simulink model "Electric"  (R2022b)
settings: Solver=VariableStepAuto  StartTime=0.0  StopTime=2  RelTol=1e-3
settings Model: Creator=Stefano  LastModifiedBy=stefanopanzieri
settings SolverCC: AlgebraicLoopSolver=TrustRegion
settings DebuggingCC: UnconnectedInputMsg=warning  UnconnectedOutputMsg=warning  UnconnectedLineMsg=warning  SFMachineParentedDataDiag=warning
settings ModelReferenceCC: EnableRefExpFcnMdlSchedulingChecks=on
settings SFSimCC: CustomCodeUndefinedFunction=UseInterfaceOnly
settings RTWCC: DLArmComputeVersion=19.05

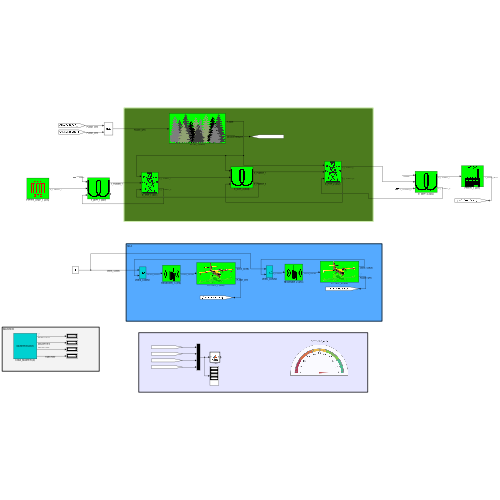
[thumbnail: Simulink's stored preview of the top-level diagram]
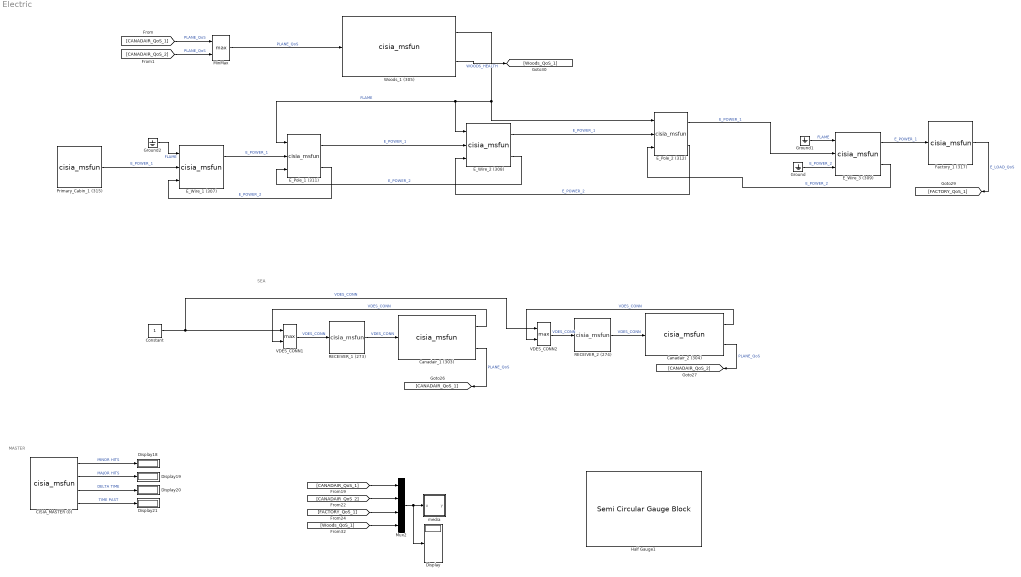
== system Electric ==
  note: SEA
  note: MASTER
  CISIA_MASTER (0) : M-S-Function  FunctionName=cisia_msfun  Parameters=Parameter1, Parameter2, Parameter3, resources, Parameter4, Parameter5, Parameter6, Parameter7, Parameter8, Parameter9,Parameter11  mask(S-function:msfcn_unit_delay){Parameter1='CISIA_MASTER', Parameter2=1, Parameter3='SistemiIoT', resources=off, Parameter4=on, Parameter5=off, Parameter6=off, Parameter7=off, Parameter8=0.001, Parameter9=off, Parameter11=on}
      mask prompts: Parameter1 "entity name"; Parameter2 "sampling time"; Parameter3 "project"; resources "Save status at each major hit"; Parameter4 "Show Operative Levels with colors"; Parameter5 "Load Entities from file"; Parameter6 "Load Start from Mask"; Parameter7 "Real Time"; Parameter8 "Real Time Hit (sec)"; Parameter9 "Skip saving"; Parameter11 "Show unconnected"
      mask help: This is a level-2 MATLAB file S-function which demonstrates CISIA entity
      mask Display: disp('MASTER BLOCK')
  Canadair_1 (303) : M-S-Function  FunctionName=cisia_msfun  Parameters=Parameter1, Parameter2, Parameter3, resources, Parameter10, codeupdate, step_received, step_computed, dynamic_computed, step_sended, id_entity, id_project, id_type, name_type, color  mask(S-function:msfcn_unit_delay){Parameter1='Canadair_1', Parameter2=1, Parameter3='', resources=|, Parameter10=off, codeupdate=off, step_received=|, step_computed=, dynamic_computed=, step_sended=|, id_entity=303, id_project=6, id_type=64, name_type=Plane, color=#FFFFFF}
      mask resources=|
      | *** INPUT RESOURCES ***
      | NUM_INPUTS 1
      | VDES_CONN (1)
      |
      | *** STATE VARIABLES ***
      | NUM_VARIABLES 3
      | Operative_Level(NUMERIC)(1)(1)
      | Mechanical_Fault(NUMERIC)(1)(0)
      | Conn_Fault(NUMERIC)(1)(0)
      |
      | *** OUTPUT RESOURCES ***
      | NUM_OUTPUTS 2
      | VDES_CONN (1)
      | PLANE_QoS (1)
      mask step_received=|
      | Conn_Fault=1-max(VDES_CONN);
      |
      |
      | Operative_Level=(1-Mechanical_Fault)*(1-Conn_Fault);
      mask step_sended=|
      | PLANE_QoS=Operative_Level;
      | VDES_CONN=1-Conn_Fault;
      mask prompts: Parameter1 "entity name"; Parameter2 "sampling time"; Parameter3 "project"; resources "input resources and state variables"; Parameter10 "Bring state variables to output"; codeupdate "update code from mask"
      mask help: This is a level-2 MATLAB file S-function which demonstrates CISIA entity
      mask DialogControl Container1 Prompt: All parameters
      mask Display: image('Icons/Canadair_1.png')
  Canadair_2 (304) : M-S-Function  FunctionName=cisia_msfun  Parameters=Parameter1, Parameter2, Parameter3, resources, Parameter10, codeupdate, step_received, step_computed, dynamic_computed, step_sended, id_entity, id_project, id_type, name_type, color  mask(S-function:msfcn_unit_delay){Parameter1='Canadair_2', Parameter2=1, Parameter3='', resources=|, Parameter10=off, codeupdate=off, step_received=|, step_computed=, dynamic_computed=, step_sended=|, id_entity=304, id_project=6, id_type=64, name_type=Plane, color=#FFFFFF}
      mask resources=|
      | *** INPUT RESOURCES ***
      | NUM_INPUTS 1
      | VDES_CONN (1)
      |
      | *** STATE VARIABLES ***
      | NUM_VARIABLES 3
      | Operative_Level(NUMERIC)(1)(1)
      | Mechanical_Fault(NUMERIC)(1)(0)
      | Conn_Fault(NUMERIC)(1)(0)
      |
      | *** OUTPUT RESOURCES ***
      | NUM_OUTPUTS 2
      | VDES_CONN (1)
      | PLANE_QoS (1)
      mask step_received=|
      | Conn_Fault=1-max(VDES_CONN);
      |
      |
      | Operative_Level=(1-Mechanical_Fault)*(1-Conn_Fault);
      mask step_sended=|
      | PLANE_QoS=Operative_Level;
      | VDES_CONN=1-Conn_Fault;
      mask prompts: Parameter1 "entity name"; Parameter2 "sampling time"; Parameter3 "project"; resources "input resources and state variables"; Parameter10 "Bring state variables to output"; codeupdate "update code from mask"
      mask help: This is a level-2 MATLAB file S-function which demonstrates CISIA entity
      mask DialogControl Container1 Prompt: All parameters
      mask Display: image('Icons/Canadair_2.png')
  Constant : Constant
  Display{,18..21} (5 alike) : Display
  E_Pole_1 (311) : M-S-Function  FunctionName=cisia_msfun  Parameters=Parameter1, Parameter2, Parameter3, resources, Parameter10, codeupdate, step_received, step_computed, dynamic_computed, step_sended, id_entity, id_project, id_type, name_type, color  mask(S-function:msfcn_unit_delay){Parameter1='E_Pole_1', Parameter2=1, Parameter3='', resources=|, Parameter10=off, codeupdate=off, step_received=|, step_computed=, dynamic_computed=, step_sended=|, id_entity=311, id_project=6, id_type=68, name_type=Electric_Pole, color=#FFFFFF}
      mask resources=|
      | *** INPUT RESOURCES ***
      | NUM_INPUTS 3
      | FLAME (1)
      | E_POWER_1 (10)
      | E_POWER_2 (10)
      |
      | *** STATE VARIABLES ***
      | NUM_VARIABLES 5
      | Operative_Level(NUMERIC)(1)(1)
      | Mechanical_Fault(NUMERIC)(1)(0)
      | Fire_Fault(NUMERIC)(1)(0)
      | Physical_Fault(NUMERIC)(1)(0)
      | Power_Gen(NUMERIC_ARRAY)(10)(0  0  0  0  0  0  0  0  0  0)
      |
      | *** OUTPUT RESOURCES ***
      | NUM_OUTPUTS 2
      | E_POWER_1 (10)
      | E_POWER_2 (10)
      mask step_received=|
      | Power_Gen=max(E_POWER_1,E_POWER_2);
      |
      | Fire_Fault=FLAME;
      |
      | Physical_Fault=max(Fire_Fault,Mechanical_Fault);
      |
      | Operative_Level=1-Physical_Fault;
      mask step_sended=|
      | E_POWER_1=Power_Gen*(1-Physical_Fault);
      | E_POWER_2=Power_Gen*(1-Physical_Fault);
      mask prompts: Parameter1 "entity name"; Parameter2 "sampling time"; Parameter3 "project"; resources "input resources and state variables"; Parameter10 "Bring state variables to output"; codeupdate "update code from mask"
      mask help: This is a level-2 MATLAB file S-function which demonstrates CISIA entity
      mask DialogControl Container1 Prompt: All parameters
      mask Display: image('Icons/Electric_Pole.png')
  E_Pole_2 (312) : M-S-Function  FunctionName=cisia_msfun  Parameters=Parameter1, Parameter2, Parameter3, resources, Parameter10, codeupdate, step_received, step_computed, dynamic_computed, step_sended, id_entity, id_project, id_type, name_type, color  mask(S-function:msfcn_unit_delay){Parameter1='E_Pole_2', Parameter2=1, Parameter3='', resources=|, Parameter10=off, codeupdate=off, step_received=|, step_computed=, dynamic_computed=, step_sended=|, id_entity=312, id_project=6, id_type=68, name_type=Electric_Pole, color=#FFFFFF}
      mask resources=|
      | *** INPUT RESOURCES ***
      | NUM_INPUTS 3
      | FLAME (1)
      | E_POWER_1 (10)
      | E_POWER_2 (10)
      |
      | *** STATE VARIABLES ***
      | NUM_VARIABLES 5
      | Operative_Level(NUMERIC)(1)(1)
      | Mechanical_Fault(NUMERIC)(1)(0)
      | Fire_Fault(NUMERIC)(1)(0)
      | Physical_Fault(NUMERIC)(1)(0)
      | Power_Gen(NUMERIC_ARRAY)(10)(0  0  0  0  0  0  0  0  0  0)
      |
      | *** OUTPUT RESOURCES ***
      | NUM_OUTPUTS 2
      | E_POWER_1 (10)
      | E_POWER_2 (10)
      mask step_received=|
      | Power_Gen=max(E_POWER_1,E_POWER_2);
      |
      | Fire_Fault=FLAME;
      |
      | Physical_Fault=max(Fire_Fault,Mechanical_Fault);
      |
      | Operative_Level=1-Physical_Fault;
      mask step_sended=|
      | E_POWER_1=Power_Gen*(1-Physical_Fault);
      | E_POWER_2=Power_Gen*(1-Physical_Fault);
      mask prompts: Parameter1 "entity name"; Parameter2 "sampling time"; Parameter3 "project"; resources "input resources and state variables"; Parameter10 "Bring state variables to output"; codeupdate "update code from mask"
      mask help: This is a level-2 MATLAB file S-function which demonstrates CISIA entity
      mask DialogControl Container1 Prompt: All parameters
      mask Display: image('Icons/Electric_Pole.png')
  E_Wire_1 (307) : M-S-Function  FunctionName=cisia_msfun  Parameters=Parameter1, Parameter2, Parameter3, resources, Parameter10, codeupdate, step_received, step_computed, dynamic_computed, step_sended, id_entity, id_project, id_type, name_type, color  mask(S-function:msfcn_unit_delay){Parameter1='E_Wire_1', Parameter2=1, Parameter3='', resources=|, Parameter10=off, codeupdate=off, step_received=|, step_computed=, dynamic_computed=, step_sended=|, id_entity=307, id_project=6, id_type=67, name_type=Electric_Wire, color=#FFFFFF}
      mask resources=|
      | *** INPUT RESOURCES ***
      | NUM_INPUTS 3
      | FLAME (1)
      | E_POWER_1 (10)
      | E_POWER_2 (10)
      |
      | *** STATE VARIABLES ***
      | NUM_VARIABLES 5
      | Operative_Level(NUMERIC)(1)(1)
      | Mechanical_Fault(NUMERIC)(1)(0)
      | Fire_Fault(NUMERIC)(1)(0)
      | Physical_Fault(NUMERIC)(1)(0)
      | Power_Gen(NUMERIC_ARRAY)(10)(0  0  0  0  0  0  0  0  0  0)
      |
      | *** OUTPUT RESOURCES ***
      | NUM_OUTPUTS 2
      | E_POWER_1 (10)
      | E_POWER_2 (10)
      mask step_received=|
      | Power_Gen=max(E_POWER_1,E_POWER_2);
      |
      | Fire_Fault=FLAME;
      |
      | Physical_Fault=max(Fire_Fault,Mechanical_Fault);
      |
      | Operative_Level=1-Physical_Fault;
      mask step_sended=|
      | E_POWER_1=Power_Gen*(1-Physical_Fault);
      | E_POWER_2=Power_Gen*(1-Physical_Fault);
      mask prompts: Parameter1 "entity name"; Parameter2 "sampling time"; Parameter3 "project"; resources "input resources and state variables"; Parameter10 "Bring state variables to output"; codeupdate "update code from mask"
      mask help: This is a level-2 MATLAB file S-function which demonstrates CISIA entity
      mask DialogControl Container1 Prompt: All parameters
      mask Display: image('Icons/Electric_Wire.png')
  E_Wire_2 (308) : M-S-Function  FunctionName=cisia_msfun  Parameters=Parameter1, Parameter2, Parameter3, resources, Parameter10, codeupdate, step_received, step_computed, dynamic_computed, step_sended, id_entity, id_project, id_type, name_type, color  mask(S-function:msfcn_unit_delay){Parameter1='E_Wire_2', Parameter2=1, Parameter3='', resources=|, Parameter10=off, codeupdate=off, step_received=|, step_computed=, dynamic_computed=, step_sended=|, id_entity=308, id_project=6, id_type=67, name_type=Electric_Wire, color=#FFFFFF}
      mask resources=|
      | *** INPUT RESOURCES ***
      | NUM_INPUTS 3
      | FLAME (1)
      | E_POWER_1 (10)
      | E_POWER_2 (10)
      |
      | *** STATE VARIABLES ***
      | NUM_VARIABLES 5
      | Operative_Level(NUMERIC)(1)(1)
      | Mechanical_Fault(NUMERIC)(1)(0)
      | Fire_Fault(NUMERIC)(1)(0)
      | Physical_Fault(NUMERIC)(1)(0)
      | Power_Gen(NUMERIC_ARRAY)(10)(0  0  0  0  0  0  0  0  0  0)
      |
      | *** OUTPUT RESOURCES ***
      | NUM_OUTPUTS 2
      | E_POWER_1 (10)
      | E_POWER_2 (10)
      mask step_received=|
      | Power_Gen=max(E_POWER_1,E_POWER_2);
      |
      | Fire_Fault=FLAME;
      |
      | Physical_Fault=max(Fire_Fault,Mechanical_Fault);
      |
      | Operative_Level=1-Physical_Fault;
      mask step_sended=|
      | E_POWER_1=Power_Gen*(1-Physical_Fault);
      | E_POWER_2=Power_Gen*(1-Physical_Fault);
      mask prompts: Parameter1 "entity name"; Parameter2 "sampling time"; Parameter3 "project"; resources "input resources and state variables"; Parameter10 "Bring state variables to output"; codeupdate "update code from mask"
      mask help: This is a level-2 MATLAB file S-function which demonstrates CISIA entity
      mask DialogControl Container1 Prompt: All parameters
      mask Display: image('Icons/Electric_Wire.png')
  E_Wire_3 (309) : M-S-Function  FunctionName=cisia_msfun  Parameters=Parameter1, Parameter2, Parameter3, resources, Parameter10, codeupdate, step_received, step_computed, dynamic_computed, step_sended, id_entity, id_project, id_type, name_type, color  mask(S-function:msfcn_unit_delay){Parameter1='E_Wire_3', Parameter2=1, Parameter3='', resources=|, Parameter10=off, codeupdate=off, step_received=|, step_computed=, dynamic_computed=, step_sended=|, id_entity=309, id_project=6, id_type=67, name_type=Electric_Wire, color=#FFFFFF}
      mask resources=|
      | *** INPUT RESOURCES ***
      | NUM_INPUTS 3
      | FLAME (1)
      | E_POWER_1 (10)
      | E_POWER_2 (10)
      |
      | *** STATE VARIABLES ***
      | NUM_VARIABLES 5
      | Operative_Level(NUMERIC)(1)(1)
      | Mechanical_Fault(NUMERIC)(1)(0)
      | Fire_Fault(NUMERIC)(1)(0)
      | Physical_Fault(NUMERIC)(1)(0)
      | Power_Gen(NUMERIC_ARRAY)(10)(0  0  0  0  0  0  0  0  0  0)
      |
      | *** OUTPUT RESOURCES ***
      | NUM_OUTPUTS 2
      | E_POWER_1 (10)
      | E_POWER_2 (10)
      mask step_received=|
      | Power_Gen=max(E_POWER_1,E_POWER_2);
      |
      | Fire_Fault=FLAME;
      |
      | Physical_Fault=max(Fire_Fault,Mechanical_Fault);
      |
      | Operative_Level=1-Physical_Fault;
      mask step_sended=|
      | E_POWER_1=Power_Gen*(1-Physical_Fault);
      | E_POWER_2=Power_Gen*(1-Physical_Fault);
      mask prompts: Parameter1 "entity name"; Parameter2 "sampling time"; Parameter3 "project"; resources "input resources and state variables"; Parameter10 "Bring state variables to output"; codeupdate "update code from mask"
      mask help: This is a level-2 MATLAB file S-function which demonstrates CISIA entity
      mask DialogControl Container1 Prompt: All parameters
      mask Display: image('Icons/Electric_Wire.png')
  Factory_1 (317) : M-S-Function  FunctionName=cisia_msfun  Parameters=Parameter1, Parameter2, Parameter3, resources, Parameter10, codeupdate, step_received, step_computed, dynamic_computed, step_sended, id_entity, id_project, id_type, name_type, color  mask(S-function:msfcn_unit_delay){Parameter1='Factory_1', Parameter2=1, Parameter3='', resources=|, Parameter10=off, codeupdate=off, step_received=|, step_computed=, dynamic_computed=, step_sended=E_LOAD_QoS=Operative_Level;, id_entity=317, id_project=6, id_type=69, name_type=Electric_Load, color=#FFFFFF}
      mask resources=|
      | *** INPUT RESOURCES ***
      | NUM_INPUTS 1
      | E_POWER_1 (10)
      |
      | *** STATE VARIABLES ***
      | NUM_VARIABLES 7
      | Operative_Level(NUMERIC)(1)(1)
      | Mechanical_Fault(NUMERIC)(1)(0)
      | Power_Fault(NUMERIC)(1)(0)
      | Fire_Fault(NUMERIC)(1)(0)
      | Physical_Fault(NUMERIC)(1)(0)
      | Power_Gen(NUMERIC_ARRAY)(10)(0  0  0  0  0  0  0  0  0  0)
      | Consumed_Power(NUMERIC_ARRAY)(10)(0  0  0  0  0  0  0  0  0  0)
      |
      | *** OUTPUT RESOURCES ***
      | NUM_OUTPUTS 1
      | E_LOAD_QoS (1)
      mask step_received=|
      | Power_Gen=max(Power_Gen_init,E_POWER_1);
      |
      | Physical_Fault=max([Fire_Fault  Mechanical_Fault] );
      |
      | Power_Fault=max(abs(Consumed_Power.*E_POWER_1-Consumed_Power));
      |
      |
      | Operative_Level=max([1-Power_Fault 0.5])*(1-Physical_Fault);
      mask prompts: Parameter1 "entity name"; Parameter2 "sampling time"; Parameter3 "project"; resources "input resources and state variables"; Parameter10 "Bring state variables to output"; codeupdate "update code from mask"
      mask help: This is a level-2 MATLAB file S-function which demonstrates CISIA entity
      mask DialogControl Container1 Prompt: All parameters
      mask Display: image('Icons/Factory_1.png')
  Ground : Ground
  Ground1 : Ground
  Ground2 : Ground
  Half Gauge1 : SemiCircularGaugeBlock  ScaleMax=1
  MinMax : MinMax  Function=max  Inputs=2
  Mux2 : Mux
  Primary_Cabin_1 (315) : M-S-Function  FunctionName=cisia_msfun  Parameters=Parameter1, Parameter2, Parameter3, resources, Parameter10, codeupdate, step_received, step_computed, dynamic_computed, step_sended, id_entity, id_project, id_type, name_type, color  mask(S-function:msfcn_unit_delay){Parameter1='Primary_Cabin_1', Parameter2=1, Parameter3='', resources=|, Parameter10=off, codeupdate=off, step_received=|, step_computed=, dynamic_computed=, step_sended=E_POWER_1=Power_Gen*(1-Physical_Fault);, id_entity=315, id_project=6, id_type=66, name_type=Electric_Plant, color=#FFFFFF}
      mask resources=|
      | *** INPUT RESOURCES ***
      | NUM_INPUTS 0
      |
      | *** STATE VARIABLES ***
      | NUM_VARIABLES 5
      | Operative_Level(NUMERIC)(1)(1)
      | Mechanical_Fault(NUMERIC)(1)(0)
      | Fire_Fault(NUMERIC)(1)(0)
      | Physical_Fault(NUMERIC)(1)(0)
      | Power_Gen(NUMERIC_ARRAY)(10)(0  0  0  0  0  0  0  0  0  0)
      |
      | *** OUTPUT RESOURCES ***
      | NUM_OUTPUTS 1
      | E_POWER_1 (10)
      mask step_received=|
      | Physical_Fault=max(Fire_Fault,Mechanical_Fault);
      |
      | Operative_Level=1-Physical_Fault;
      mask prompts: Parameter1 "entity name"; Parameter2 "sampling time"; Parameter3 "project"; resources "input resources and state variables"; Parameter10 "Bring state variables to output"; codeupdate "update code from mask"
      mask help: This is a level-2 MATLAB file S-function which demonstrates CISIA entity
      mask DialogControl Container1 Prompt: All parameters
      mask Display: image('Icons/Primary_Cabin_1.png')
  RECEIVER_1 (273) : M-S-Function  FunctionName=cisia_msfun  Parameters=Parameter1, Parameter2, Parameter3, resources, Parameter10, codeupdate, step_received, step_computed, dynamic_computed, step_sended, id_entity, id_project, id_type, name_type, color  mask(S-function:msfcn_unit_delay){Parameter1='RECEIVER_1', Parameter2=1, Parameter3='', resources=|, Parameter10=off, codeupdate=off, step_received=Conn_Fault=1-VDES_CONN;, step_computed=, dynamic_computed=, step_sended=VDES_CONN=1-Conn_Fault;, id_entity=273, id_project=6, id_type=59, name_type=VDES_RECEIVER, color=#FFFFFF}
      mask resources=|
      | *** INPUT RESOURCES ***
      | NUM_INPUTS 1
      | VDES_CONN (1)
      |
      | *** STATE VARIABLES ***
      | NUM_VARIABLES 3
      | Operative_Level(NUMERIC)(1)(1)
      | Connection(NUMERIC_ARRAY)(20)(0  0  0  0  0  0  0  0  0  0  0  0  0  0  0  0  0  0  0  0)
      | Conn_Fault(NUMERIC)(1)(0)
      |
      | *** OUTPUT RESOURCES ***
      | NUM_OUTPUTS 1
      | VDES_CONN (1)
      mask prompts: Parameter1 "entity name"; Parameter2 "sampling time"; Parameter3 "project"; resources "input resources and state variables"; Parameter10 "Bring state variables to output"; codeupdate "update code from mask"
      mask help: This is a level-2 MATLAB file S-function which demonstrates CISIA entity
      mask DialogControl Container1 Prompt: All parameters
      mask Display: image('Icons/VDES_RECEIVER.png')
  RECEIVER_2 (274) : M-S-Function  FunctionName=cisia_msfun  Parameters=Parameter1, Parameter2, Parameter3, resources, Parameter10, codeupdate, step_received, step_computed, dynamic_computed, step_sended, id_entity, id_project, id_type, name_type, color  mask(S-function:msfcn_unit_delay){Parameter1='RECEIVER_2', Parameter2=1, Parameter3='', resources=|, Parameter10=off, codeupdate=off, step_received=Conn_Fault=1-VDES_CONN;, step_computed=, dynamic_computed=, step_sended=VDES_CONN=1-Conn_Fault;, id_entity=274, id_project=6, id_type=59, name_type=VDES_RECEIVER, color=#FFFFFF}
      mask resources=|
      | *** INPUT RESOURCES ***
      | NUM_INPUTS 1
      | VDES_CONN (1)
      |
      | *** STATE VARIABLES ***
      | NUM_VARIABLES 3
      | Operative_Level(NUMERIC)(1)(1)
      | Connection(NUMERIC_ARRAY)(20)(0  0  0  0  0  0  0  0  0  0  0  0  0  0  0  0  0  0  0  0)
      | Conn_Fault(NUMERIC)(1)(0)
      |
      | *** OUTPUT RESOURCES ***
      | NUM_OUTPUTS 1
      | VDES_CONN (1)
      mask prompts: Parameter1 "entity name"; Parameter2 "sampling time"; Parameter3 "project"; resources "input resources and state variables"; Parameter10 "Bring state variables to output"; codeupdate "update code from mask"
      mask help: This is a level-2 MATLAB file S-function which demonstrates CISIA entity
      mask DialogControl Container1 Prompt: All parameters
      mask Display: image('Icons/VDES_RECEIVER.png')
  VDES_CONN1 : MinMax  Function=max  Inputs=2
  VDES_CONN2 : MinMax  Function=max  Inputs=2
  Woods_1 (305) : M-S-Function  FunctionName=cisia_msfun  Parameters=Parameter1, Parameter2, Parameter3, resources, Parameter10, codeupdate, step_received, step_computed, dynamic_computed, step_sended, id_entity, id_project, id_type, name_type, color  mask(S-function:msfcn_unit_delay){Parameter1='Woods_1', Parameter2=1, Parameter3='SistemiIoT', resources=|, Parameter10=off, codeupdate=off, step_received=|, step_computed=, dynamic_computed=, step_sended=|, id_entity=305, id_project=6, id_type=65, name_type=Forest, color=#FFFFFF}
      mask resources=|
      | *** INPUT RESOURCES ***
      | NUM_INPUTS 1
      | PLANE_QoS (1)
      |
      | *** STATE VARIABLES ***
      | NUM_VARIABLES 2
      | Operative_Level(NUMERIC)(1)(1)
      | Fire_Fault(NUMERIC)(1)(0)
      |
      | *** OUTPUT RESOURCES ***
      | NUM_OUTPUTS 2
      | FLAME (1)
      | WOODS_HEALTH (1)
      mask step_received=|
      | Operative_Level=(1-Fire_Fault)*max(PLANE_QoS, 0.5);
      |
      | WOODS_HEALTH=Operative_Level;
      mask step_sended=|
      | FLAME=Fire_Fault;
      | WOODS_HEALTH=Operative_Level;
      mask prompts: Parameter1 "entity name"; Parameter2 "sampling time"; Parameter3 "project"; resources "input resources and state variables"; Parameter10 "Bring state variables to output"; codeupdate "update code from mask"
      mask help: This is a level-2 MATLAB file S-function which demonstrates CISIA entity
      mask DialogControl Container1 Prompt: All parameters
      mask Display: image('Icons/Forest.png')
  media : MATLAB Function  TreatAsAtomicUnit=on
  wires:
  RECEIVER_1 (273)/1 -> Canadair_1 (303)/1  "VDES_CONN"
  RECEIVER_2 (274)/1 -> Canadair_2 (304)/1  "VDES_CONN"
  VDES_CONN2/1 -> RECEIVER_2 (274)/1  "VDES_CONN"
  VDES_CONN1/1 -> RECEIVER_1 (273)/1  "VDES_CONN"
  Canadair_2 (304)/1 -> VDES_CONN2/2  "VDES_CONN"
  Canadair_1 (303)/1 -> VDES_CONN1/2  "VDES_CONN"
  Canadair_2 (304)/2 -> [CANADAIR_QoS_2]  "PLANE_QoS"
  Canadair_1 (303)/2 -> [CANADAIR_QoS_1]  "PLANE_QoS"
  E_Wire_3 (309)/1 -> Factory_1 (317)/1  "E_POWER_1"
  Factory_1 (317)/1 -> [FACTORY_QoS_1]  "E_LOAD_QoS"
  Woods_1 (305)/1 -> E_Wire_2 (308)/1, E_Pole_1 (311)/1, E_Pole_2 (312)/1  "FLAME"
  E_Pole_1 (311)/1 -> E_Wire_2 (308)/2  "E_POWER_1"
  E_Wire_2 (308)/1 -> E_Pole_2 (312)/2  "E_POWER_1"
  E_Pole_2 (312)/1 -> E_Wire_3 (309)/2  "E_POWER_1"
  Ground/1 -> E_Wire_3 (309)/3  "E_POWER_2"
  Ground1/1 -> E_Wire_3 (309)/1  "FLAME"
  Ground2/1 -> E_Wire_1 (307)/1  "FLAME"
  E_Pole_2 (312)/2 -> E_Wire_2 (308)/3  "E_POWER_2"
  E_Wire_2 (308)/2 -> E_Pole_1 (311)/3  "E_POWER_2"
  E_Wire_1 (307)/1 -> E_Pole_1 (311)/2  "E_POWER_1"
  E_Pole_1 (311)/2 -> E_Wire_1 (307)/3  "E_POWER_2"
  Primary_Cabin_1 (315)/1 -> E_Wire_1 (307)/2  "E_POWER_1"
  Woods_1 (305)/2 -> [Woods_QoS_1]  "WOODS_HEALTH"
  E_Wire_3 (309)/2 -> E_Pole_2 (312)/3  "E_POWER_2"
  [Woods_QoS_1] -> Mux2/4
  [FACTORY_QoS_1] -> Mux2/3
  Mux2/1 -> media/1(u), Display/1
  [CANADAIR_QoS_1] -> Mux2/1
  [CANADAIR_QoS_2] -> Mux2/2
  Constant/1 -> VDES_CONN2/1, VDES_CONN1/1  "VDES_CONN"
  MinMax/1 -> Woods_1 (305)/1  "PLANE_QoS"
  [CANADAIR_QoS_1] -> MinMax/1  "PLANE_QoS"
  [CANADAIR_QoS_2] -> MinMax/2  "PLANE_QoS"
  CISIA_MASTER (0)/2 -> Display19/1  "MAJOR HITS"
  CISIA_MASTER (0)/4 -> Display21/1  "TIME PAST"
  CISIA_MASTER (0)/3 -> Display20/1  "DELTA TIME"
  CISIA_MASTER (0)/1 -> Display18/1  "MINOR HITS"

== matlab function Electric/media ==
  data: u input; y output
function y = media(u)

y = mean(u);
